simulink model "PI_controller_sim"  (R2024b)
settings: Solver=VariableStepAuto  StartTime=0.0  StopTime=10.0  RelTol=1e-3
values from neighbouring files (symbols this model uses):
  m = 1400    [mpc3.m]    (also in prueba_mpc.m; prueba_mpc2.m)
settings Model: Creator=inaki  LastModifiedBy=inaki

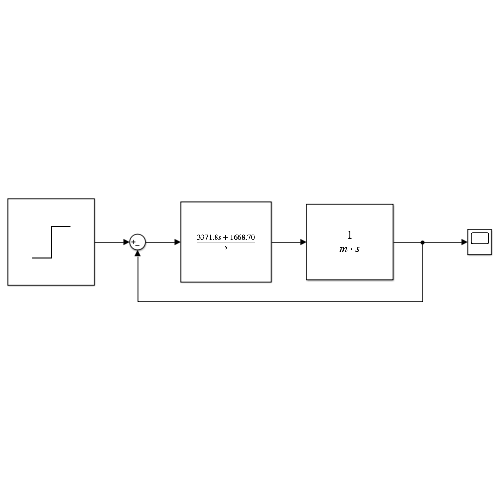
[thumbnail: Simulink's stored preview of the top-level diagram]
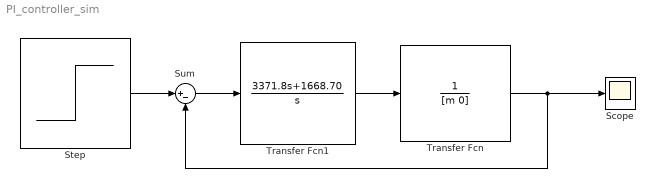
== system PI_controller_sim ==
  Scope : Scope
  Step : Step  After=5  SampleTime=0
  Sum : Sum  Inputs=|+-
  Transfer Fcn : TransferFcn  Denominator=[m 0]
  Transfer Fcn1 : TransferFcn  Numerator=[3371.8 1668.70]  Denominator=[1 0]
  wires:
  Step/1 -> Sum/1
  Sum/1 -> Transfer Fcn1/1
  Transfer Fcn1/1 -> Transfer Fcn/1
  Transfer Fcn/1 -> Sum/2, Scope/1
